simulink model "motorsAdry"  (R2019a)
settings: Solver=VariableStepAuto  StartTime=0.0  StopTime=50  RelTol=1e-3
values from neighbouring files (symbols this model uses):
  a = randi(200)    [motorsArchivo.m]
  b = randi(250)    [motorsArchivo.m]
  tDisCol = e + 2    [motorsArchivo.m]
  tDisCol2 = tDisCol + 40    [motorsArchivo.m]
  tDisCol3 = tDisCol2 + e + 2    [motorsArchivo.m]
  tDisFi = d+2    [motorsArchivo.m]
  tDisFi2 = tDisFi +2    [motorsArchivo.m]
  tDisFi3 = tDisFi2 +round(5/2.25+1)+2    [motorsArchivo.m]
  tDisHeat = d + 2    [motorsArchivo.m]
  tDisHeat2 = tDisHeat + 60    [motorsArchivo.m]
  tDisHeat3 = tDisHeat2 + d + 2    [motorsArchivo.m]
  tDisPack = e + 2    [motorsArchivo.m]
  tDisPack2 = tDisPack + 60    [motorsArchivo.m]
  tDisPack3 = tDisPack2 + e + 2    [motorsArchivo.m]
  tF = tVer3 +  round(25/(0.5*2.25) + 1)+2    [motorsArchivo.m]
  tF2 = tF + round(100/2.25 +1 )    [motorsArchivo.m]
  tHor = round(a/2.25 + 1)    [motorsArchivo.m]
  tHor2 = tPla2 + round(100/2.25 + 1)+1    [motorsArchivo.m]
  tPla = tVer + round(40/(0.5*2.25) + 1)+1    [motorsArchivo.m]
  tPla2 = tPla + round(40/(0.5*2.25) + 1)+2    [motorsArchivo.m]
  tPla3 = tVer2 + round(25/(0.5*2.25) + 1)+1    [motorsArchivo.m]
  tVer = tHor + round(b/(2*2.25) + 1)    [motorsArchivo.m]
  tVer2 = tHor2 +round(125/(2*2.25) + 1)+1    [motorsArchivo.m]
  tVer3 = tPla3 + round(1/(2*2.25) + 1)+2    [motorsArchivo.m]
libraries: cstblocks x12
settings Model: Creator=Dell  LastModifiedBy=Dell

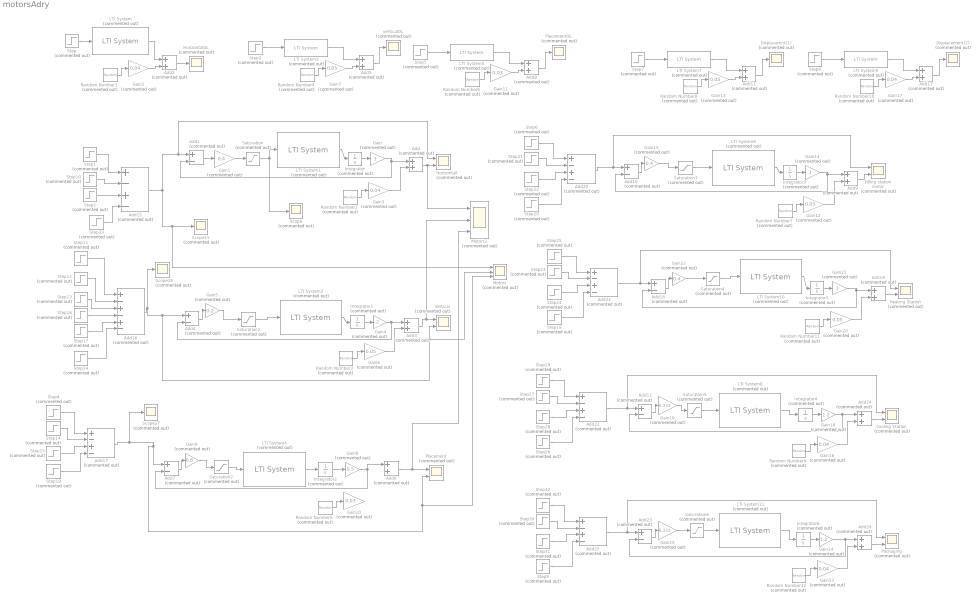
== system motorsAdry ==
  Add{,2..3,5..6,8..9,11,13..14,19,24} (12 alike) : Sum  Commented=on
  Add{1,4,7,10,12,18,23} (7 alike) : Sum  Commented=on  Inputs=+-
  Add{15,17,20..22,25} (6 alike) : Sum  Commented=on  Inputs=+-+-
  Add16 : Sum  Commented=on  Inputs=+-+-+-
  Cooling Station : Scope  Commented=on  NumInputPorts=2
  Displacement(2) : Scope  Commented=on
  Displacemnt(1) : Scope  Commented=on
  Filling station motor : Scope  Commented=on  NumInputPorts=2
  Gain : Gain  Commented=on
  Gain1 : Gain  Commented=on  Gain=0.4
  Gain10 : Gain  Commented=on  Gain=0.03
  Gain11 : Gain  Commented=on  Gain=0.03
  Gain{6..7,12..13,20} (5 alike) : Gain  Commented=on  Gain=0.05
  Gain14 : Gain  Commented=on
  Gain15 : Gain  Commented=on  Gain=0.4
  Gain{2..3,16..17,23} (5 alike) : Gain  Commented=on  Gain=0.04
  Gain18 : Gain  Commented=on  Gain=1.2
  Gain19 : Gain  Commented=on  Gain=0.333
  Gain21 : Gain  Commented=on
  Gain22 : Gain  Commented=on  Gain=0.4
  Gain24 : Gain  Commented=on  Gain=1.2
  Gain25 : Gain  Commented=on  Gain=0.333
  Gain4 : Gain  Commented=on  Gain=2
  Gain5 : Gain  Commented=on  Gain=0.2
  Gain8 : Gain  Commented=on  Gain=0.5
  Gain9 : Gain  Commented=on  Gain=0.8
  Heating Station : Scope  Commented=on  NumInputPorts=2
  HorizontalOL : Scope  Commented=on
  "Horizontall " : Scope  Commented=on  NumInputPorts=2
  Integrator{,1..6} (7 alike) : Integrator  Commented=on
  LTI System{,1..11} (12 alike) : cstblocks/LTI System  Commented=on  sys=tf(22.846,[1 3.023 9.139])  IC=[]
  Motors : Scope  Commented=on  NumInputPorts=3
  Motors1 : Scope  Commented=on  NumInputPorts=3
  Packaging : Scope  Commented=on  NumInputPorts=2
  Placement : Scope  Commented=on  NumInputPorts=2
  PlacementOL : Scope  Commented=on
  Random Number{1..12} (12 alike) : RandomNumber  Commented=on  SampleTime=0.01
  Saturation{,1..6} (7 alike) : Saturate  Commented=on  UpperLimit=0.9  LowerLimit=-0.9
  Scope{,15..17} (4 alike) : Scope  Commented=on
  Step{,3,5,7,9} (5 alike) : Step  Commented=on  Time=0  SampleTime=0
  Step1 : Step  Commented=on  Time=0  After=a  SampleTime=0
  Step10 : Step  Commented=on  Time=tPla2  After=a  SampleTime=0
  Step11 : Step  Commented=on  Time=tHor+1  After=b  SampleTime=0
  Step12 : Step  Commented=on  Time=tHor2  After=b  SampleTime=0
  Step13 : Step  Commented=on  Time=tHor2  After=125  SampleTime=0
  Step14 : Step  Commented=on  Time=tPla  After=40  SampleTime=0
  Step15 : Step  Commented=on  Time=tVer2  After=25  SampleTime=0
  Step16 : Step  Commented=on  Time=tPla3  After=125  SampleTime=0
  Step17 : Step  Commented=on  Time=tPla3  After=124  SampleTime=0
  Step18 : Step  Commented=on  Time=tVer3  After=25  SampleTime=0
  Step19 : Step  Commented=on  Time=tDisHeat3  After=30  SampleTime=0
  Step2 : Step  Commented=on  Time=tPla2  After=100  SampleTime=0
  Step20 : Step  Commented=on  Time=tDisFi3  After=30  SampleTime=0
  Step21 : Step  Commented=on  Time=tDisFi  After=30  SampleTime=0
  Step22 : Step  Commented=on  Time=tDisFi2  After=30  SampleTime=0
  Step23 : Step  Commented=on  Time=tDisHeat  After=30  SampleTime=0
  Step24 : Step  Commented=on  Time=tDisHeat2  After=30  SampleTime=0
  Step{6,25,29,32} (4 alike) : Step  Commented=on  Time=0  After=30  SampleTime=0
  Step26 : Step  Commented=on  Time=tDisCol3  After=30  SampleTime=0
  Step27 : Step  Commented=on  Time=tDisCol  After=30  SampleTime=0
  Step28 : Step  Commented=on  Time=tDisCol2  After=30  SampleTime=0
  Step30 : Step  Commented=on  Time=tDisPack  After=30  SampleTime=0
  Step31 : Step  Commented=on  Time=tDisPack2  After=30  SampleTime=0
  Step33 : Step  Commented=on  Time=tF  After=100  SampleTime=0
  Step34 : Step  Commented=on  Time=tF2  After=124  SampleTime=0
  Step4 : Step  Commented=on  Time=tVer  After=40  SampleTime=0
  Step8 : Step  Commented=on  Time=tDisPack3  After=30  SampleTime=0
  Vertical : Scope  Commented=on  NumInputPorts=2
  verticalOL : Scope  Commented=on
  wires:
  Step/1 -> LTI System/1
  Add15/1 -> "Horizontall "/1, Add1/1, Motors/1, Scope15/1
  LTI System1/1 -> Integrator/1
  Integrator/1 -> Gain/1
  Gain/1 -> Add1/2, Add/1
  Add/1 -> Motors1/1, "Horizontall "/2
  Add2/1 -> HorizontalOL/1
  LTI System/1 -> Add2/1
  Gain2/1 -> Add2/2
  Random Number1/1 -> Gain2/1
  Random Number2/1 -> Gain3/1
  Random Number3/1 -> Gain6/1
  Gain5/1 -> Saturation1/1
  Gain4/1 -> Add4/2, Add3/1
  Add4/1 -> Gain5/1
  Integrator1/1 -> Gain4/1
  LTI System2/1 -> Integrator1/1
  Add5/1 -> verticalOL/1
  Random Number4/1 -> Gain7/1
  LTI System3/1 -> Add5/1
  Step3/1 -> LTI System3/1
  Gain7/1 -> Add5/2
  Gain6/1 -> Add3/2
  LTI System4/1 -> Integrator2/1
  Gain11/1 -> Add8/2
  Step5/1 -> LTI System5/1
  LTI System5/1 -> Add8/1
  Random Number6/1 -> Gain11/1
  Add8/1 -> PlacementOL/1
  Gain8/1 -> Add6/1, Add7/2
  Random Number5/1 -> Gain10/1
  Integrator2/1 -> Gain8/1
  Add7/1 -> Gain9/1
  Random Number8/1 -> Gain13/1
  LTI System7/1 -> Add11/1
  Step7/1 -> LTI System7/1
  Gain13/1 -> Add11/2
  Add20/1 -> Filling station motor/1, Add10/1
  LTI System6/1 -> Integrator3/1
  Add11/1 -> Displacemnt(1)/1
  Gain12/1 -> Add9/2
  Add10/1 -> Gain15/1
  Gain14/1 -> Add10/2, Add9/1
  Integrator3/1 -> Gain14/1
  Random Number7/1 -> Gain12/1
  Integrator4/1 -> Gain18/1
  Gain18/1 -> Add12/2, Add14/1
  Random Number9/1 -> Gain16/1
  Add12/1 -> Gain19/1
  Gain16/1 -> Add14/2
  Add13/1 -> Displacement(2)/1
  LTI System8/1 -> Integrator4/1
  Add22/1 -> Cooling Station/1, Add12/1
  Gain17/1 -> Add13/2
  Random Number10/1 -> Gain17/1
  Step9/1 -> LTI System9/1
  LTI System9/1 -> Add13/1
  Add14/1 -> Cooling Station/2
  Step1/1 -> Add15/1
  Step11/1 -> Add16/1
  Step4/1 -> Add17/1
  Add3/1 -> Motors1/2, Vertical/1
  Add6/1 -> Motors1/3, Placement/1
  Integrator5/1 -> Gain21/1
  Add18/1 -> Gain22/1
  Gain20/1 -> Add19/2
  Add19/1 -> Heating Station/2
  Add21/1 -> Heating Station/1, Add18/1
  LTI System10/1 -> Integrator5/1
  Random Number11/1 -> Gain20/1
  Gain21/1 -> Add18/2, Add19/1
  Step22/1 -> Add20/3
  Step6/1 -> Add20/1
  Step21/1 -> Add20/2
  Step20/1 -> Add20/4
  Step24/1 -> Add21/3
  Step23/1 -> Add21/2
  Step25/1 -> Add21/1
  Step19/1 -> Add21/4
  Step27/1 -> Add22/2
  Step29/1 -> Add22/1
  Step28/1 -> Add22/3
  Step26/1 -> Add22/4
  Add24/1 -> Packaging/2
  Gain23/1 -> Add24/2
  Integrator6/1 -> Gain24/1
  Random Number12/1 -> Gain23/1
  LTI System11/1 -> Integrator6/1
  Add23/1 -> Gain25/1
  Gain24/1 -> Add23/2, Add24/1
  Step8/1 -> Add25/4
  Step31/1 -> Add25/3
  Step32/1 -> Add25/1
  Add25/1 -> Packaging/1, Add23/1
  Step30/1 -> Add25/2
  Add1/1 -> Gain1/1
  Add17/1 -> Scope17/1, Add7/1, Motors/3, Placement/2
  Add16/1 -> Vertical/2, Motors/2, Add4/1, Scope16/1
  Saturation/1 -> Scope/1, LTI System1/1
  Gain1/1 -> Saturation/1
  Gain3/1 -> Add/2
  Saturation1/1 -> LTI System2/1
  Saturation2/1 -> LTI System4/1
  Gain9/1 -> Saturation2/1
  Step14/1 -> Add17/2
  Step10/1 -> Add15/2
  Step2/1 -> Add15/3
  Step12/1 -> Add16/2
  Step13/1 -> Add16/3
  Step17/1 -> Add16/5
  Step33/1 -> Add15/4
  Step34/1 -> Add16/6
  Step15/1 -> Add17/3
  Step16/1 -> Add16/4
  Step18/1 -> Add17/4
  Gain15/1 -> Saturation3/1
  Saturation3/1 -> LTI System6/1
  Add9/1 -> Filling station motor/2
  Gain22/1 -> Saturation4/1
  Saturation4/1 -> LTI System10/1
  Gain19/1 -> Saturation5/1
  Saturation5/1 -> LTI System8/1
  Saturation6/1 -> LTI System11/1
  Gain25/1 -> Saturation6/1
